simulink model "model_input_output"  (R2019b)
settings: Solver=VariableStepAuto  StartTime=0.0  StopTime=500.0  RelTol=1e-3
settings Model: Creator=rafa  LastModifiedBy=rafa

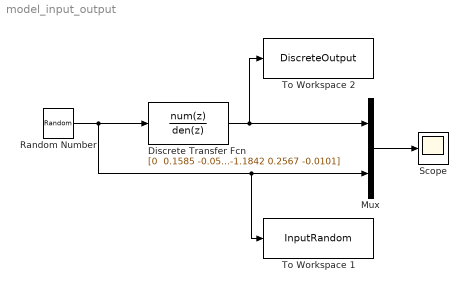
== system model_input_output ==
  "Discrete Transfer Fcn " : DiscreteTransferFcn  Numerator="[0  0.1585 -0.0558 -0.0246]"  Denominator=[1.0000 -1.1842 0.2567 -0.0101]
  Mux : Mux  Inputs=2
  "Random Number " : RandomNumber  SampleTime=1
  "Scope " : Scope
  To Workspace 1 : ToWorkspace  VariableName=InputRandom  SampleTime=-1
  To Workspace 2 : ToWorkspace  VariableName=DiscreteOutput  SampleTime=-1
  wires:
  "Random Number "/1 -> To Workspace 1/1, Mux/2, "Discrete Transfer Fcn "/1
  Mux/1 -> "Scope "/1
  "Discrete Transfer Fcn "/1 -> To Workspace 2/1, Mux/1
